simulink model "GH2_vent_prop_valve_tuner"  (R2024b)
settings: Solver=ode15s  StartTime=0.0  StopTime=300  RelTol=1e-3
settings Model: Creator=MW  LastModifiedBy=MW

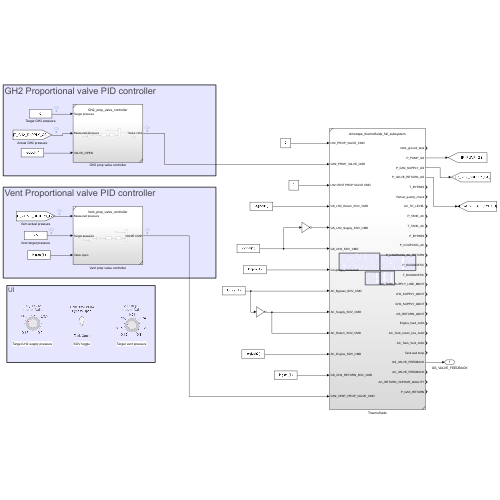
[thumbnail: Simulink's stored preview of the top-level diagram]
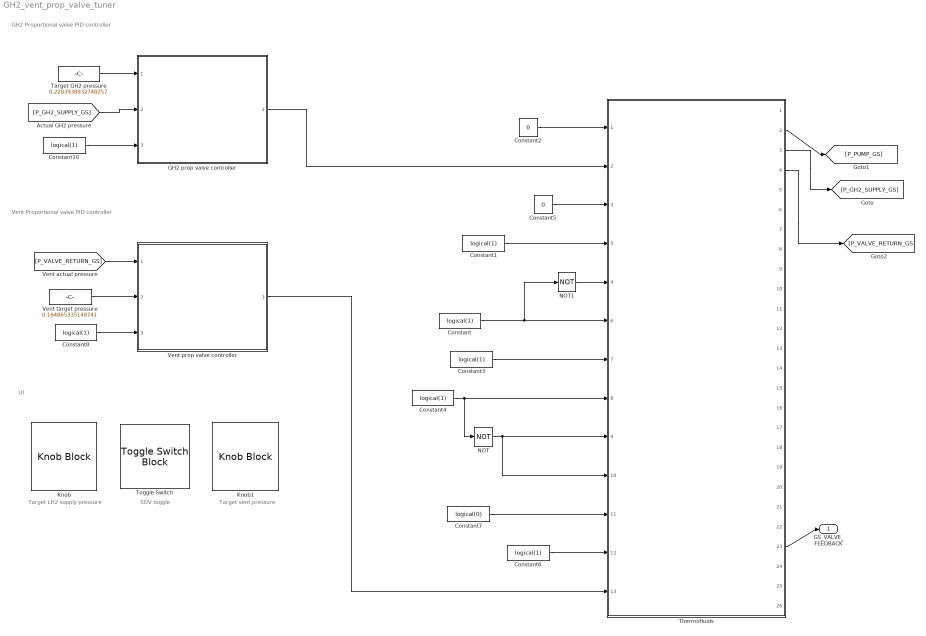
== system GH2_vent_prop_valve_tuner ==
  note: Target LH2 supply pressure
  note: UI
  note: Target vent pressure
  note: SOV toggle
  note: Vent Proportional valve PID controller
  note: GH2 Proportional valve PID controller
  Constant{,1,3..4,6,8,10} (7 alike) : Constant  Value=logical(1)
  Constant2 : Constant  Value=0
  Constant5 : Constant  Value=0
  Constant7 : Constant  Value=logical(0)
  GH2 prop valve controller : Subsystem  ReferencedSubsystem=GH2_prop_valve_controller
  Knob : KnobBlock  ScaleMin=0.12  ScaleMax=0.5
  Knob1 : KnobBlock  ScaleMin=0.12  ScaleMax=0.3
  NOT : Logic  Operator=NOT  IconShape=distinctive  AllPortsSameDT=off  OutDataTypeStr=boolean
  NOT1 : Logic  Operator=NOT  IconShape=distinctive  AllPortsSameDT=off  OutDataTypeStr=boolean
  Target GH2 pressure : Constant  Value=0.2283938932748257
  Thermofluids : Subsystem  ReferencedSubsystem=simscape_thermofluids_full_subsystem
      settings: PortSchema="{\"entries\":[{\"content\":{\"sides\":[{\"content\":{\"connectorIds\":[\"In1\",\"In2\",\"In3\",\"In5\",\"In4\",\"In6\",\"In7\",\"In8\",\"In9\",\"In10\",\"In11\",\"In12\",\"In13\"]},\"type\":\"ConnectorPlacement.EquallySpacedRectSide\",\"uuid\":\"0abe1c09-fd1c-4f21-adb2-1ba1f178e40f\"},{\"content\":{\"connectorIds\":[\"Out1\",\"Out2\",\"Out3\",\"Out4\",\"Out5\",\"Out6\",\"Out7\",\"Out8\",\"Out9\",\"Out10\",\"Out11\",\"Out12\",\"Out13\",\"Out14\",\"Out15\",\"Out16\",\"Out17\",\"Out18\",\"Out19\",\"Out20\",\"Out21\",\"Out22\",\"Out23\",\"Out24\",\"Out25\",\"Out26\"],\"side\":\"RIGHT\"},\"type\":\"ConnectorPlacement.EquallySpacedRectSide\",\"uuid\":\"d1a7e852-e313-42b4-9b52-713a379b8745\"},{\"content\":{\"side\":\"TOP\"},\"type\":\"ConnectorPlacement.EquallySpacedRectSide\",\"uuid\":\"bcf0416b-035c-45e3-b36d-7b1188a80ffd\"}]},\"type\":\"ConnectorPlacement.EquallySpacedConnector\",\"uuid\":\"eb213e55-2670-4e0e-a421-e9d6b5e6eb19\"}],\"packageUris\":[\"http://schema.mathworks.com/mf0/Connector/R2020b\"],\"version\":\"1.0\"}"
  Toggle Switch : ToggleSwitchBlock
      settings: Values={{'Tank Open', 'Bypass Open'}, [0 1]}
  Vent prop valve controller : Subsystem  ReferencedSubsystem=Vent_prop_valve_controller
  Vent target pressure : Constant  Value=0.164865335148741
  GS_VALVE_FEEDBACK : Outport
  wires:
  Constant1/1 -> Thermofluids/5
  Constant3/1 -> Thermofluids/7
  Constant4/1 -> NOT/1, Thermofluids/8
  NOT/1 -> Thermofluids/10, Thermofluids/9
  Constant7/1 -> Thermofluids/11
  Thermofluids/3 -> [P_GH2_SUPPLY_GS]
  Thermofluids/2 -> [P_PUMP_GS]
  Vent target pressure/1 -> Vent prop valve controller/2
  Thermofluids/4 -> [P_VALVE_RETURN_GS]
  [P_VALVE_RETURN_GS] -> Vent prop valve controller/1
  NOT1/1 -> Thermofluids/4
  Constant/1 -> Thermofluids/6, NOT1/1
  Constant8/1 -> Vent prop valve controller/3
  [P_GH2_SUPPLY_GS] -> GH2 prop valve controller/2
  Target GH2 pressure/1 -> GH2 prop valve controller/1
  Constant10/1 -> GH2 prop valve controller/3
  GH2 prop valve controller/1 -> Thermofluids/2
  Constant2/1 -> Thermofluids/1
  Constant5/1 -> Thermofluids/3
  Vent prop valve controller/1 -> Thermofluids/13
  Constant6/1 -> Thermofluids/12
  Thermofluids/23 -> GS_VALVE_FEEDBACK/1
